simulink model "ASMC"  (R2015a)
settings: Solver=ode45  SolverMode=SingleTasking  StartTime=0.0  StopTime=10.0  RelTol=1e-3
values from neighbouring files (symbols this model uses):
  anpha_0 = 5    [ANN_params.m]    (also in furuta.m)
  J0 = 4.4*10^(-3)    (= 0.0044)    [ANN_params.m]    (also in furuta.m)
  J1 = 5.5026*10^(-4)    (= 0.00055026)    [ANN_params.m]    (also in furuta.m)
  kd = 0.35    [ANN_params.m]
  L0 = 0.157    [ANN_params.m]    (also in furuta.m)
  L1 = 0.133    [ANN_params.m]    (also in furuta.m)
  m1 = 0.078    [ANN_params.m]    (also in furuta.m = 0.0933)
  theta_0 = 0    [ANN_params.m]    (also in furuta.m)
undefined symbols (not defined in the file or in its folder): k1, phi, theta
settings Model: CovMetricSettings=dwe  CovHtmlReporting=off  covSaveCumulativeToWorkspaceVar=off  CovSaveSingleToWorkspaceVar=off  CovExternalEMLEnable=on  Creator=Chechao  LastModifiedBy=chech
settings SolverCC: MaxConsecutiveMinStep=10
settings DataIOCC: LimitDataPoints=off  SaveFormat=Dataset
settings DebuggingCC: SFUnexpectedBacktrackingDiag=error  SFNoUnconditionalDefaultTransitionDiag=error
settings HardwareCC: ProdBitPerPointer=64  ProdLargestAtomicFloat=Float  ProdIntDivRoundTo=Zero  ProdEndianess=LittleEndian  ProdHWDeviceType=Specified
settings ModelReferenceCC: PropagateSignalLabelsOutOfModel=on
settings GRTTargetCC: TargetLangStandard=C99 (ISO)  GeneratePreprocessorConditionals=Use local settings
settings ConfigurationSet: Description=Simscape Multibody
settings ExplorerConfigSet: InternalSimMechanicsExplorerSettings="<ExplorerConfiguration><canonicalview>planar_xy</canonicalview><AnimationSetting><BasePlaybackSpeed>1.0</BasePlaybackSpeed><PlaybackSpeedFactor>1.0</PlaybackSpeedFactor></AnimationSetting><TilePanel><TileInfo><Tiles Columns=\"1\" Count=\"1\" Rows=\"1\"><Column Left=\"2\" Weight=\"1\"/><Column Left=\"815\"/><Row Top=\"2\" Weight=\"1\"/><Row Top=\"278\"/><Tile Height=\"1\" Width=\"1\" X=\"0\" Y=\"0\"/></Tiles></TileInfo><SceneInfo><SceneViewer><BGColor><R>0.60000002384185791</R><G>0.60000002384185791</G><B>0.60000002384185791</B></BGColor><Camera><DoPerspective>off</DoPerspective><Position><X>3.0348189574883895</X><Y>0.89503316987109838</Y><Z>1.1148954709131602</Z></Position><Center><X>1.4216968578267744</X><Y>0.23812580067611089</Y><Z>-0.36954855728247171</Z></Center><Up><X>-0.074382553953715444</X><Y>0.93933115277276391</Y><Z>-0.3348495499443197</Z></Up><ViewLimDist>1</ViewLimDist><YLim>1.1431212443461942</YLim><XLim>3.4422077919638205</XLim></Camera></SceneViewer></SceneInfo></TilePanel><MechEditorPanel><Cameras/><GfxPanelCameraMap/><VideoCreator><PlaybackSpeedRatio>1.0</PlaybackSpeedRatio><FrameRate>30</FrameRate><VideoFormat>Motion JPEG AVI</VideoFormat><FrameSize>auto</FrameSize></VideoCreator></MechEditorPanel></ExplorerConfiguration>"

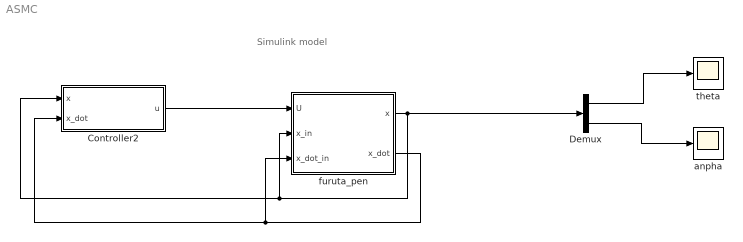
== system ASMC ==
  note: Simulink model
  Controller2 : Subsystem
  Demux : Demux  Outputs=2
  anpha : Scope
      settings: YMin=-0.30589  YMax=0.44831
  furuta_pen : Subsystem
  theta : Scope
      settings: ShowLegends=on  YMin=-1.89166  YMax=17.02491
  wires:
  furuta_pen/2(x_dot) -> Controller2/2(x_dot), furuta_pen/3(x_dot_in)
  furuta_pen/1(x) -> Demux/1, Controller2/1(x), furuta_pen/2(x_in)
  Controller2/1(u) -> furuta_pen/1(U)
  Demux/1 -> theta/1
  Demux/2 -> anpha/1

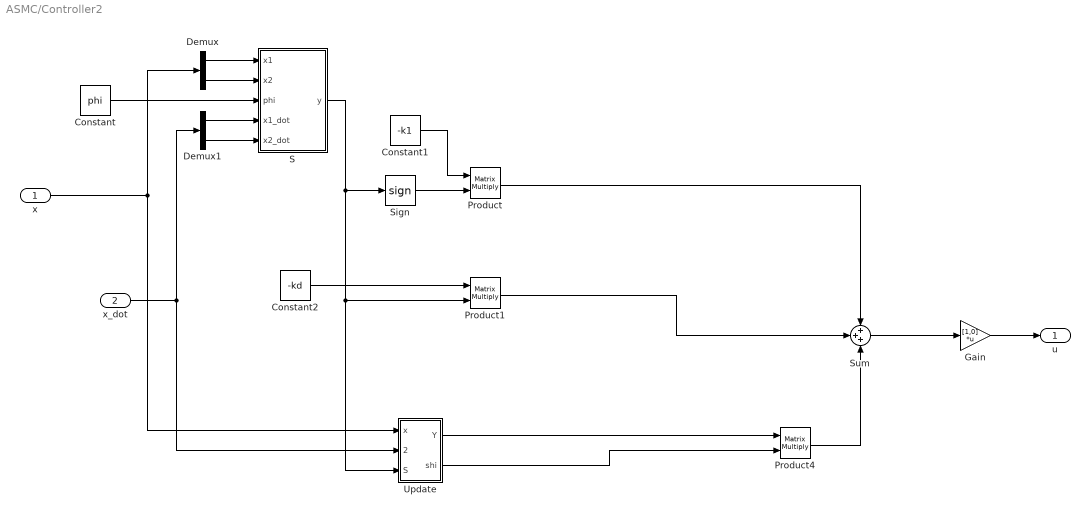
== system ASMC/Controller2 ==
  x : Inport
  x_dot : Inport  Port=2
  Constant : Constant  Value=phi
  Constant1 : Constant  Value=-k1
  Constant2 : Constant  Value=-kd
  Demux : Demux  Outputs=2
  Demux1 : Demux  Outputs=2
  Gain : Gain  Gain=[1,0]  Multiplication=Matrix(K*u)
  Product : Product  Multiplication=Matrix(*)
  Product1 : Product  Multiplication=Matrix(*)
  Product4 : Product  Multiplication=Matrix(*)
  S : MATLAB Function  TreatAsAtomicUnit=on
  Sign : Signum
  Sum : Sum  Inputs=3
  Update : Subsystem
  u : Outport
  wires:
  x/1 -> Demux/1, Update/1(x)
  x_dot/1 -> Update/2(x_dot), Demux1/1
  S/1(y) -> Update/3(S), Product1/2, Sign/1
  Sign/1 -> Product/2
  Constant1/1 -> Product/1
  Constant2/1 -> Product1/1
  Product/1 -> Sum/1
  Product1/1 -> Sum/2
  Product4/1 -> Sum/3
  Sum/1 -> Gain/1
  Update/1(Y) -> Product4/1
  Update/2(shi) -> Product4/2
  Demux/1 -> S/1(x1)
  Demux/2 -> S/2(x2)
  Demux1/1 -> S/4(x1_dot)
  Demux1/2 -> S/5(x2_dot)
  Constant/1 -> S/3(phi)
  Gain/1 -> u/1

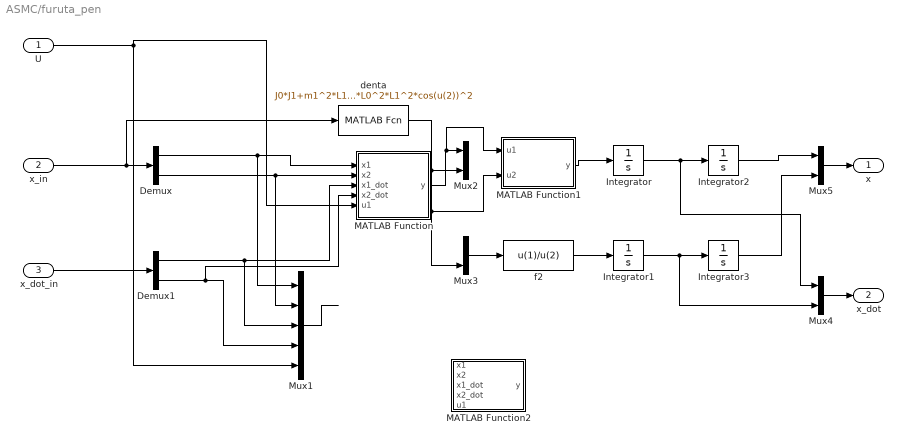
== system ASMC/furuta_pen ==
  U : Inport
  x_in : Inport  Port=2
  x_dot_in : Inport  Port=3
  Demux : Demux  Outputs=2
  Demux1 : Demux  Outputs=2
  Integrator : Integrator
  Integrator1 : Integrator
  Integrator2 : Integrator  InitialCondition=theta_0*pi/180
  Integrator3 : Integrator  InitialCondition=anpha_0/180*pi
  MATLAB Function : MATLAB Function  TreatAsAtomicUnit=on
  MATLAB Function1 : MATLAB Function  TreatAsAtomicUnit=on
  MATLAB Function2 : MATLAB Function  TreatAsAtomicUnit=on
  Mux1 : Mux  Inputs=5
  Mux{2..5} (4 alike) : Mux  Inputs=2
  denta : MATLABFcn  MATLABFcn=J0*J1+m1^2*L1^4*sin(u(2))^2+m1^2*L0^2*L1^2+J0*m1*L1^2+J1*m1*L0^2+J1*m1*L1^2*sin(u(2))^2-m1^2*L0^2*L1^2*cos(u(2))^2
  f2 : MATLABFcn  MATLABFcn=u(1)/u(2)
  x : Outport
  x_dot : Outport  Port=2
  wires:
  x_in/1 -> Demux/1, denta/1
  Mux1/1 -> ?
  Mux3/1 -> f2/1
  ? -> Mux3/1
  MATLAB Function1/1(y) -> Integrator/1
  f2/1 -> Integrator1/1
  Integrator/1 -> Mux4/1, Integrator2/1
  Integrator1/1 -> Mux4/2, Integrator3/1
  Mux4/1 -> x_dot/1
  Mux5/1 -> x/1
  Integrator2/1 -> Mux5/1
  Integrator3/1 -> Mux5/2
  x_dot_in/1 -> Demux1/1
  Demux/1 -> MATLAB Function/1(x1), Mux1/1
  Demux/2 -> MATLAB Function/2(x2), Mux1/2
  Demux1/2 -> MATLAB Function/4(x2_dot), Mux1/4
  Demux1/1 -> MATLAB Function/3(x1_dot), Mux1/3
  U/1 -> Mux1/5, MATLAB Function/5(u1)
  MATLAB Function/1(y) -> MATLAB Function1/1(u1), Mux2/1
  denta/1 -> Mux2/2, MATLAB Function1/2(u2), Mux3/2

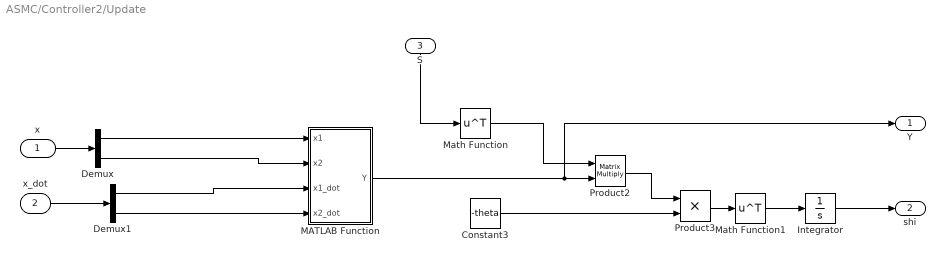
== system ASMC/Controller2/Update ==
  x : Inport
  x_dot : Inport  Port=2
  S : Inport  Port=3
  Constant3 : Constant  Value=-theta
  Demux : Demux  Outputs=2
  Demux1 : Demux  Outputs=2
  Integrator : Integrator  InitialCondition=[0;0;0]
  MATLAB Function : MATLAB Function  TreatAsAtomicUnit=on
  Math Function : Math  Operator=transpose  SaturateOnIntegerOverflow=on
  Math Function1 : Math  Operator=transpose  SaturateOnIntegerOverflow=on
  Product2 : Product  Multiplication=Matrix(*)
  Product3 : Product
  Y : Outport
  shi : Outport  Port=2
  wires:
  Integrator/1 -> shi/1
  S/1 -> Math Function/1
  Product3/1 -> Math Function1/1
  MATLAB Function/1(Y) -> Y/1, Product2/2
  Constant3/1 -> Product3/2
  Math Function/1 -> Product2/1
  Product2/1 -> Product3/1
  x/1 -> Demux/1
  Demux/1 -> MATLAB Function/1(x1)
  Demux/2 -> MATLAB Function/2(x2)
  Demux1/1 -> MATLAB Function/3(x1_dot)
  Demux1/2 -> MATLAB Function/4(x2_dot)
  x_dot/1 -> Demux1/1
  Math Function1/1 -> Integrator/1

== matlab function ASMC/Controller2/Update/MATLAB Function ==
  data: x1 input; Y output; x2 input; x1_dot input; x2_dot input
function Y = Y(x1,x2,x1_dot,x2_dot)
%#codegen
%x1 = x(1);
%x2 = x(2);
%x1_dot = x_dot(1);
%x2_dot = x_dot(2);
Y = [x1,x1_dot,0;
    x2,x2_dot,sin(x2)];

== matlab function ASMC/Controller2/S ==
  data: x1 input; x2 input; phi input; y output; x1_dot input; x2_dot input
function y = S(x1,x2,phi,x1_dot,x2_dot)
%#codegen
y = -[x1_dot;x2_dot]-phi*[x1;x2];

== matlab function ASMC/furuta_pen/MATLAB Function ==
  data: x1 input; y output; x2 input; x1_dot input; x2_dot input; u1 input
function y = fcn(x1,x2,x1_dot,x2_dot,u1)
%#codegen
m1=0.078;
L0=0.157;
L1=0.133;
J0=4.4*10^(-3);
J1=5.5026*10^(-4);
beta0 = 5.8*10^(-4);
beta1 = 1.4142*10^(-3);
g = 9.81;
u = [x1,x2,x1_dot,x2_dot,u1];
y = m1*L0*L1*cos(u(2))*(0.5*m1*L1^2*sin(2*u(2))*u(3)^2+m1*g*L1*sin(u(2))-beta1*u(4))-(m1*L1^2+J1)*(m1*L1^2*sin(2*u(2))*u(3)*u(4)+m1*L0*L1*sin(u(2))*u(4)^2-u(5)+beta0*u(3));

== matlab function ASMC/furuta_pen/MATLAB Function1 ==
  data: u1 input; y output; u2 input
function y = fcn(u1,u2)
%#codegen

y = u1/u2;

== matlab function ASMC/furuta_pen/MATLAB Function2 ==
  data: x1 input; y output; x2 input; x1_dot input; x2_dot input; u1 input
function y = fcn(x1,x2,x1_dot,x2_dot,u1)
%#codegen
m1=0.078;
L0=0.157;
L1=0.133;
J0=4.4*10^(-3);
J1=5.5026*10^(-4);
beta0 = 5.8*10^(-4);
beta1 = 1.4142*10^(-3);
g = 9.81;
u = [x1,x2,x1_dot,x2_dot,u1];
y = (m1*L0^2+m1*L1^2*sin(u(2))^2+J0)*(0.5*m1*L1^2*sin(2*u(2))*u(3)^2+m1*g*L1*sin(u(2))-beta1*u(4))-m1*L0*L1*cos(u(2))*(m1*L1^2*sin(2*u(2))*u(3)*u(4)+m1*L0*L1*sin(u(2))*u(4)^2-u(5)+beta0*u(3));
